simulink subsystem "Controls_ThorneFleissner"  (R2020b)
settings: Solver=VariableStepAuto  StartTime=0.0  StopTime=10.0  RelTol=1e-3
libraries: simulink_extras x3
settings Model: Creator=rthom  LastModifiedBy=rthom

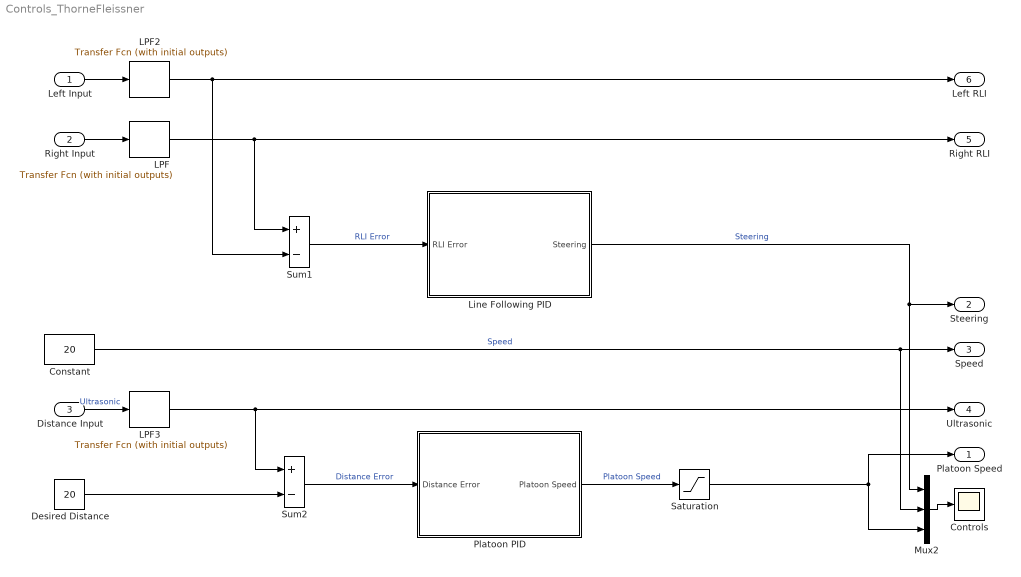
== system Controls_ThorneFleissner ==
  Left Input : Inport
  Right Input : Inport  Port=2
  Distance Input : Inport  Port=3
  Constant : Constant  Value=20
  Controls : Scope
  Desired Distance : Constant  Value=20
  LPF : simulink_extras/Additional Linear/Transfer Fcn (with initial outputs)  N=[1]  D="[0.02  1]"  Y0=0  U0=0
  LPF2 : simulink_extras/Additional Linear/Transfer Fcn (with initial outputs)  N=[1]  D="[0.02  1]"  Y0=0  U0=0
  LPF3 : simulink_extras/Additional Linear/Transfer Fcn (with initial outputs)  N=[1]  D="[0.02  1]"  Y0=0  U0=0
  Line Following PID : Subsystem
  Mux2 : Mux  Inputs=3
  Platoon PID : Subsystem
  Saturation : Saturate  UpperLimit=30  LowerLimit=0
  Sum1 : Sum  Inputs=+-
  Sum2 : Sum  Inputs=+-
  Platoon Speed : Outport
  Steering : Outport  Port=2
  Speed : Outport  Port=3
  Ultrasonic : Outport  Port=4
  Right RLI : Outport  Port=5
  Left RLI : Outport  Port=6
  wires:
  LPF2/1 -> Left RLI/1, Sum1/2
  Constant/1 -> Speed/1, Mux2/2  "Speed"
  Mux2/1 -> Controls/1
  Right Input/1 -> LPF/1
  LPF/1 -> Right RLI/1, Sum1/1
  Left Input/1 -> LPF2/1
  Distance Input/1 -> LPF3/1  "Ultrasonic"
  Desired Distance/1 -> Sum2/2
  LPF3/1 -> Ultrasonic/1, Sum2/1
  Platoon PID/1(Platoon Speed) -> Saturation/1  "Platoon Speed"
  Sum2/1 -> Platoon PID/1(Distance Error)  "Distance Error"
  Line Following PID/1(Steering) -> Steering/1, Mux2/1  "Steering"
  Sum1/1 -> Line Following PID/1(RLI Error)  "RLI Error"
  Saturation/1 -> Platoon Speed/1, Mux2/3

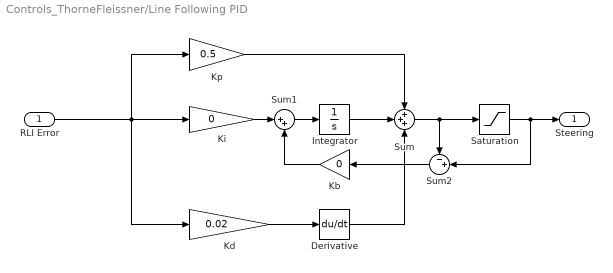
== system Controls_ThorneFleissner/Line Following PID ==
  RLI Error : Inport
  Derivative : Derivative
  Integrator : Integrator
  Kb : Gain  Gain=0
  Kd : Gain  Gain=0.02
  Ki : Gain  Gain=0
  Kp : Gain  Gain=0.5
  Saturation : Saturate  UpperLimit=15  LowerLimit=-15
  Sum : Sum  Inputs=+++
  Sum1 : Sum  Inputs=|++
  Sum2 : Sum  Inputs=-+|
  Steering : Outport
  wires:
  Sum2/1 -> Kb/1
  Kb/1 -> Sum1/2
  Sum1/1 -> Integrator/1
  Ki/1 -> Sum1/1
  Saturation/1 -> Steering/1, Sum2/2
  Derivative/1 -> Sum/3
  RLI Error/1 -> Kp/1, Ki/1, Kd/1
  Integrator/1 -> Sum/2
  Kp/1 -> Sum/1
  Kd/1 -> Derivative/1
  Sum/1 -> Saturation/1, Sum2/1

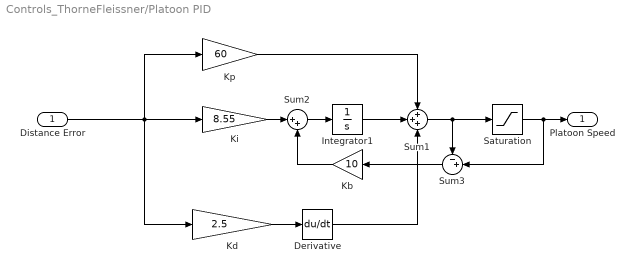
== system Controls_ThorneFleissner/Platoon PID ==
  Distance Error : Inport
  Derivative : Derivative
  Integrator1 : Integrator
  Kb : Gain  Gain=10
  Kd : Gain  Gain=2.5
  Ki : Gain  Gain=8.55
  Kp : Gain  Gain=60
  Saturation : Saturate  UpperLimit=30  LowerLimit=0
  Sum1 : Sum  Inputs=+++
  Sum2 : Sum  Inputs=|++
  Sum3 : Sum  Inputs=-+|
  Platoon Speed : Outport
  wires:
  Kp/1 -> Sum1/1
  Derivative/1 -> Sum1/3
  Ki/1 -> Sum2/1
  Sum1/1 -> Saturation/1, Sum3/1
  Integrator1/1 -> Sum1/2
  Sum3/1 -> Kb/1
  Kb/1 -> Sum2/2
  Saturation/1 -> Sum3/2, Platoon Speed/1
  Sum2/1 -> Integrator1/1
  Distance Error/1 -> Kp/1, Kd/1, Ki/1
  Kd/1 -> Derivative/1
